simulink model "V10MODE_TEST"  (R2020b)
settings: Solver=VariableStepAuto  StartTime=0.0  StopTime=10.0  RelTol=1e-3
values from neighbouring files (symbols this model uses):
  HD = 180/pi    (= 57.2957795131)    [mode_data.m]
undefined symbols (not defined in the file or in its folder): Vehicle
libraries: sharedutil x2
settings Model: Creator=a4327481  LastModifiedBy=a4327481

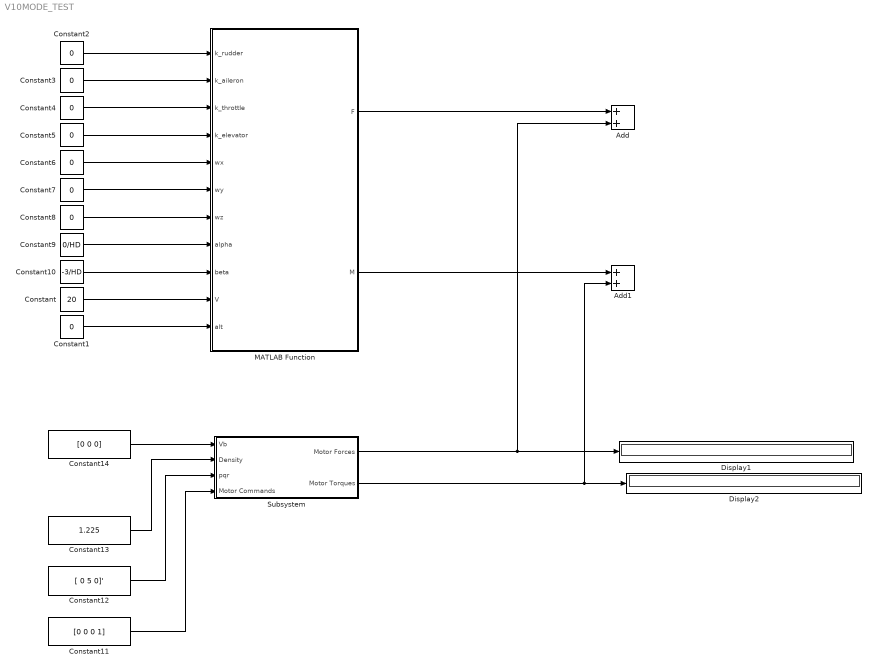
== system V10MODE_TEST ==
  Add : Sum
  Add1 : Sum
  Constant : Constant  Value=20
  Constant{1..8} (8 alike) : Constant  Value=0
  Constant10 : Constant  Value=-3/HD
  Constant11 : Constant  Value=[0 0 0 1]  VectorParams1D=off
  Constant12 : Constant  Value=[ 0 5 0]'
  Constant13 : Constant  Value=1.225
  Constant14 : Constant  Value=[0 0 0]
  Constant9 : Constant  Value=0/HD
  Display1 : Display
  Display2 : Display
  MATLAB Function : MATLAB Function  TreatAsAtomicUnit=on
  Subsystem : Subsystem
  wires:
  Constant/1 -> MATLAB Function/10(V)
  Constant1/1 -> MATLAB Function/11(alt)
  Constant2/1 -> MATLAB Function/1(k_rudder)
  Constant3/1 -> MATLAB Function/2(k_aileron)
  Constant4/1 -> MATLAB Function/3(k_throttle)
  Constant5/1 -> MATLAB Function/4(k_elevator)
  Constant6/1 -> MATLAB Function/5(wx)
  Constant7/1 -> MATLAB Function/6(wy)
  Constant8/1 -> MATLAB Function/7(wz)
  Constant10/1 -> MATLAB Function/9(beta)
  Constant9/1 -> MATLAB Function/8(alpha)
  Constant11/1 -> Subsystem/4(Motor Commands)
  Constant12/1 -> Subsystem/3(pqr)
  Constant13/1 -> Subsystem/2(Density)
  Constant14/1 -> Subsystem/1(Vb)
  MATLAB Function/1(F) -> Add/1
  MATLAB Function/2(M) -> Add1/1
  Subsystem/2(Motor Torques) -> Display2/1, Add1/2
  Subsystem/1(Motor Forces) -> Add/2, Display1/1

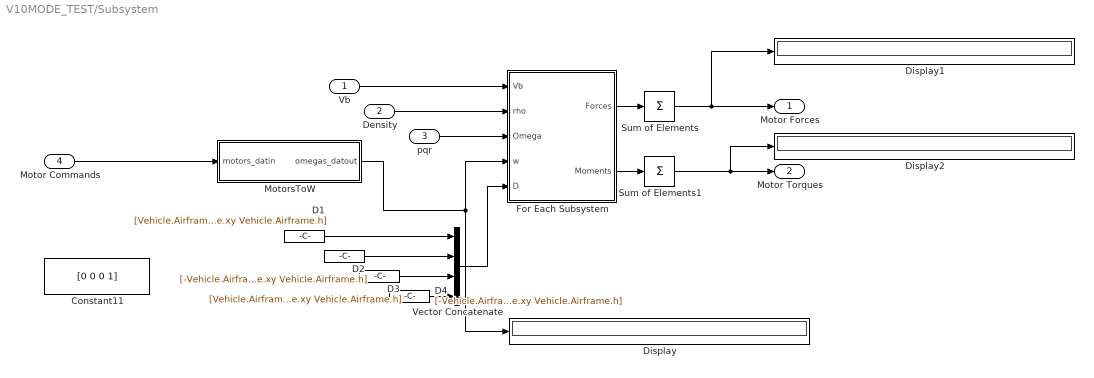
== system V10MODE_TEST/Subsystem ==
  Vb : Inport
  Density : Inport  Port=2
  pqr : Inport  Port=3
  Motor Commands : Inport  Port=4
  Constant11 : Constant  Value=[0 0 0 1]  VectorParams1D=off
  D1 : Constant  Value=[Vehicle.Airframe.xy +Vehicle.Airframe.xy Vehicle.Airframe.h]
  D2 : Constant  Value=[-Vehicle.Airframe.xy -Vehicle.Airframe.xy Vehicle.Airframe.h]
  D3 : Constant  Value=[Vehicle.Airframe.xy -Vehicle.Airframe.xy Vehicle.Airframe.h]
  D4 : Constant  Value=[-Vehicle.Airframe.xy Vehicle.Airframe.xy Vehicle.Airframe.h]
  Display : Display
  Display1 : Display
  Display2 : Display
  For Each Subsystem : Subsystem  TreatAsAtomicUnit=on
  MotorsToW : Subsystem
  Sum of Elements : Sum  Inputs=+  CollapseMode=Specified dimension  CollapseDim=2
  Sum of Elements1 : Sum  Inputs=+  CollapseMode=Specified dimension  CollapseDim=2
  Vector Concatenate : Concatenate  NumInputs=4  Mode=Multidimensional array  ConcatenateDimension=2
  Motor Forces : Outport  Unit=N  VectorParamsAs1DForOutWhenUnconnected=off
  Motor Torques : Outport  Port=2  Unit=N*m  VectorParamsAs1DForOutWhenUnconnected=off
  wires:
  Vector Concatenate/1 -> For Each Subsystem/5(D)
  Density/1 -> For Each Subsystem/2(rho)
  D4/1 -> Vector Concatenate/4
  Vb/1 -> For Each Subsystem/1(Vb)
  Sum of Elements1/1 -> Motor Torques/1, Display2/1
  D3/1 -> Vector Concatenate/3
  Sum of Elements/1 -> Motor Forces/1, Display1/1
  pqr/1 -> For Each Subsystem/3(Omega)
  D1/1 -> Vector Concatenate/1
  For Each Subsystem/2(Moments) -> Sum of Elements1/1
  For Each Subsystem/1(Forces) -> Sum of Elements/1
  D2/1 -> Vector Concatenate/2
  MotorsToW/1(omegas_datout) -> For Each Subsystem/4(w), Display/1
  Motor Commands/1 -> MotorsToW/1(motors_datin)

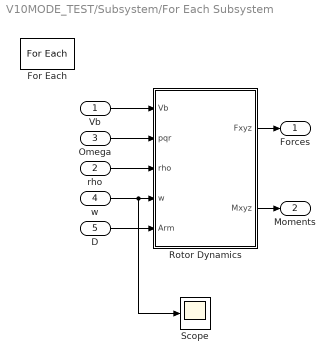
== system V10MODE_TEST/Subsystem/For Each Subsystem ==
  Vb : Inport  PortDimensions=3
  rho : Inport  Port=2  PortDimensions=1
  Omega : Inport  Port=3
  w : Inport  Port=4  Partition=on  PartitionDimension=2  PartitionWidth=1  PartitionOffset=0
  D : Inport  Port=5  Partition=on  PartitionDimension=2  PartitionWidth=1  PartitionOffset=0
  For Each : ForEach  DisableCoverage=on
  Rotor Dynamics : Subsystem  AncestorBlock=dynamicsLibrary/Rotor Dynamics  TreatAsAtomicUnit=on
      mask init:
      | aeroicon('aeroblk');
      settings: RTWFcnNameOpts=Use subsystem name  RTWFileNameOpts=Use function name
  Scope : Scope
  Forces : Outport  ConcatenationDimension=2  VectorParamsAs1DForOutWhenUnconnected=off
  Moments : Outport  Port=2  ConcatenationDimension=2  VectorParamsAs1DForOutWhenUnconnected=off
  wires:
  Rotor Dynamics/1(Fxyz) -> Forces/1
  Rotor Dynamics/2(Mxyz) -> Moments/1
  Vb/1 -> Rotor Dynamics/1(Vb)
  Omega/1 -> Rotor Dynamics/2(pqr)
  rho/1 -> Rotor Dynamics/3(rho)
  D/1 -> Rotor Dynamics/5(Arm)
  w/1 -> Scope/1, Rotor Dynamics/4(w)

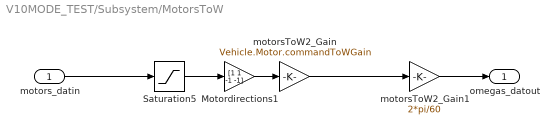
== system V10MODE_TEST/Subsystem/MotorsToW ==
  motors_datin : Inport
  Motordirections1 : Gain  Gain=[1 1 -1 -1]  ParamDataTypeStr=single  OutDataTypeStr=Inherit: Inherit via back propagation  SaturateOnIntegerOverflow=on
  Saturation5 : Saturate  UpperLimit=1  LowerLimit=realmin  OutDataTypeStr=Inherit: Inherit via back propagation
  motorsToW2_Gain : Gain  Gain=Vehicle.Motor.commandToWGain  ParamDataTypeStr=single  OutDataTypeStr=Inherit: Inherit via back propagation  SaturateOnIntegerOverflow=on
  motorsToW2_Gain1 : Gain  Gain=2*pi/60  ParamDataTypeStr=single  OutDataTypeStr=Inherit: Inherit via back propagation  SaturateOnIntegerOverflow=on
  omegas_datout : Outport  VectorParamsAs1DForOutWhenUnconnected=off
  wires:
  Saturation5/1 -> Motordirections1/1
  Motordirections1/1 -> motorsToW2_Gain/1
  motors_datin/1 -> Saturation5/1
  motorsToW2_Gain/1 -> motorsToW2_Gain1/1
  motorsToW2_Gain1/1 -> omegas_datout/1

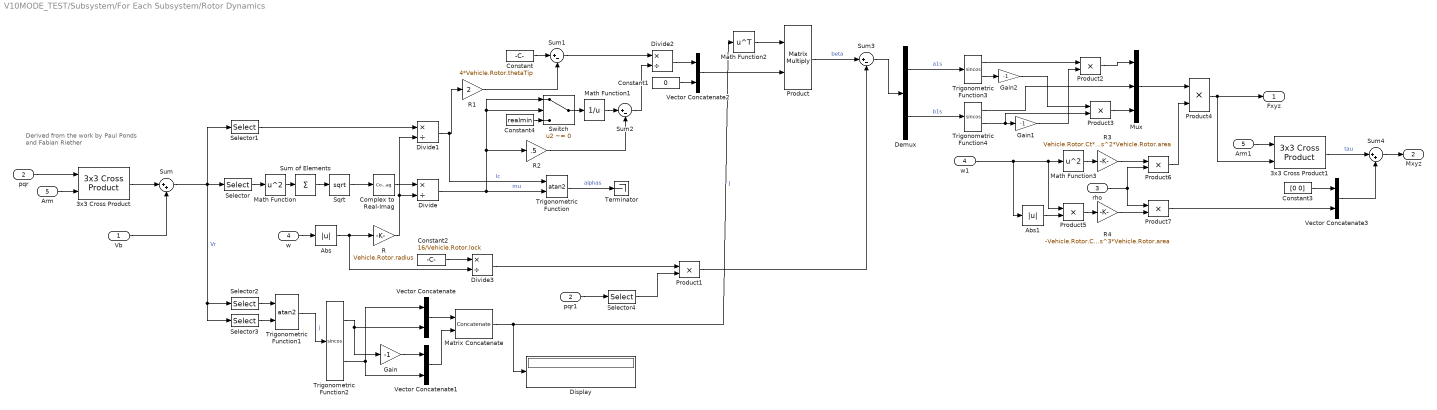
== system V10MODE_TEST/Subsystem/For Each Subsystem/Rotor Dynamics ==
  note: Derived from the work by Paul Ponds
      | and Fabian Riether
  Vb : Inport  PortDimensions=3
  pqr : Inport  Port=2  PortDimensions=3
  rho : Inport  Port=3  PortDimensions=1
  w : Inport  Port=4  PortDimensions=[1 1]
  Arm : Inport  Port=5  PortDimensions=[3 1]
  3x3 Cross Product : sharedutil/3x3 Cross Product  aMode=aMode
      settings: SourceProductBaseCode=AE,PW,MT,UV,VE,VP
  3x3 Cross Product1 : sharedutil/3x3 Cross Product  aMode=aMode
      settings: SourceProductBaseCode=AE,PW,MT,UV,VE,VP
  Abs : Abs
  Abs1 : Abs
  Arm1 : InportShadow  Port=5  PortDimensions=[3 1]
  Complex to Real-Imag : ComplexToRealImag  Output=Real
  Constant : Constant  Value=4*Vehicle.Rotor.thetaTip
  Constant1 : Constant  Value=0
  Constant2 : Constant  Value=16/Vehicle.Rotor.lock
  Constant3 : Constant  Value=[0 0]
  Constant4 : Constant  Value=realmin
  Demux : Demux  Outputs=2
  Display : Display
  Divide{,1..3} (4 alike) : Product  Inputs=*/
  Gain : Gain  Gain=-1
  Gain1 : Gain  Gain=-1
  Gain2 : Gain  Gain=-1
  Math Function : Math  Operator=square  SignedPower=on  SaturateOnIntegerOverflow=on
  Math Function1 : Math  Operator=reciprocal  SignedPower=on  SaturateOnIntegerOverflow=on
  Math Function2 : Math  Operator=transpose  SignedPower=on  SaturateOnIntegerOverflow=on
  Math Function3 : Math  Operator=square  SignedPower=on  SaturateOnIntegerOverflow=on
  Matrix Concatenate : Concatenate  Mode=Multidimensional array  ConcatenateDimension=2
  Mux : Mux  Inputs=3
  Product : Product  Multiplication=Matrix(*)
  Product{1..7} (7 alike) : Product
  R : Gain  Gain=Vehicle.Rotor.radius
  R1 : Gain  Gain=2
  R2 : Gain  Gain=.5
  R3 : Gain  Gain=Vehicle.Rotor.Ct*Vehicle.Rotor.radius^2*Vehicle.Rotor.area
  R4 : Gain  Gain=-Vehicle.Rotor.Cq*Vehicle.Rotor.radius^3*Vehicle.Rotor.area
  Selector : Selector  InputPortWidth=3  IndexOptions=Index vector (dialog)  Indices=[1 2]  OutputSizes=1
  Selector1 : Selector  InputPortWidth=3  IndexOptions=Index vector (dialog)  Indices=[3]  OutputSizes=1
  Selector2 : Selector  InputPortWidth=3  IndexOptions=Index vector (dialog)  Indices=[2]  OutputSizes=1
  Selector3 : Selector  InputPortWidth=3  IndexOptions=Index vector (dialog)  Indices=[1]  OutputSizes=1
  Selector4 : Selector  InputPortWidth=3  IndexOptions=Index vector (dialog)  Indices=[2 1]  OutputSizes=1
  Sqrt : Sqrt  OutputSignalType=complex  SaturateOnIntegerOverflow=on
  Sum : Sum  Inputs=|++
  Sum of Elements : Sum  Inputs=+
  Sum1 : Sum  Inputs=|+-
  Sum2 : Sum  Inputs=|+-
  Sum3 : Sum  Inputs=|+-
  Sum4 : Sum  Inputs=|++
  Switch : Switch  Criteria=u2 ~= 0
  Terminator : Terminator
  Trigonometric Function : Trigonometry  Operator=atan2
  Trigonometric Function1 : Trigonometry  Operator=atan2
  Trigonometric Function2 : Trigonometry  Operator=sincos
  Trigonometric Function3 : Trigonometry  Operator=sincos
  Trigonometric Function4 : Trigonometry  Operator=sincos
  Vector Concatenate{,1..3} (4 alike) : Concatenate
  pqr1 : InportShadow  Port=2  PortDimensions=3
  w1 : InportShadow  Port=4  PortDimensions=[1 1]
  Fxyz : Outport  PortDimensions=[3 1]  VectorParamsAs1DForOutWhenUnconnected=off
  Mxyz : Outport  Port=2  PortDimensions=[3 1]  VectorParamsAs1DForOutWhenUnconnected=off
  wires:
  Complex to Real-Imag/1 -> Divide/1
  Sqrt/1 -> Complex to Real-Imag/1
  Constant4/1 -> Switch/3
  Switch/1 -> Math Function1/1
  Product1/1 -> Sum3/2
  rho/1 -> Product7/1, Product6/2
  Product7/1 -> Vector Concatenate3/2
  Product6/1 -> Product4/2
  Sum4/1 -> Mxyz/1
  3x3 Cross Product1/1 -> Sum4/1  "tau"
  Product4/1 -> Fxyz/1, 3x3 Cross Product1/2
  Arm1/1 -> 3x3 Cross Product1/1
  Vector Concatenate3/1 -> Sum4/2
  Constant3/1 -> Vector Concatenate3/1
  R4/1 -> Product7/2
  Product5/1 -> R4/1
  Abs1/1 -> Product5/2
  R3/1 -> Product6/1
  Mux/1 -> Product4/1
  Gain2/1 -> Product3/1
  Product3/1 -> Mux/3
  Trigonometric Function3/2 -> Gain2/1
  Trigonometric Function4/1 -> Mux/2
  Product2/1 -> Mux/1
  Trigonometric Function3/1 -> Product2/1
  Gain1/1 -> Product2/2
  Trigonometric Function4/2 -> Gain1/1, Product3/2
  Demux/2 -> Trigonometric Function4/1  "b1s"
  Demux/1 -> Trigonometric Function3/1  "a1s"
  Sum3/1 -> Demux/1
  Math Function3/1 -> R3/1
  w1/1 -> Math Function3/1, Product5/1, Abs1/1
  Divide3/1 -> Product1/1
  Abs/1 -> R/1, Divide3/2
  Selector4/1 -> Product1/2
  pqr1/1 -> Selector4/1
  Constant2/1 -> Divide3/1
  Product/1 -> Sum3/1  "beta"
  Math Function2/1 -> Product/1
  Vector Concatenate2/1 -> Product/2
  Constant1/1 -> Vector Concatenate2/2
  Divide2/1 -> Vector Concatenate2/1
  Sum2/1 -> Divide2/2
  R2/1 -> Sum2/2
  Math Function1/1 -> Sum2/1
  Sum1/1 -> Divide2/1
  R1/1 -> Sum1/2
  Constant/1 -> Sum1/1
  Matrix Concatenate/1 -> Display/1, Math Function2/1  "J"
  Vector Concatenate1/1 -> Matrix Concatenate/2
  Vector Concatenate/1 -> Matrix Concatenate/1
  Trigonometric Function2/1 -> Gain/1, Vector Concatenate/2
  Gain/1 -> Vector Concatenate1/1
  Trigonometric Function2/2 -> Vector Concatenate/1, Vector Concatenate1/2
  Trigonometric Function1/1 -> Trigonometric Function2/1  "j"
  Selector3/1 -> Trigonometric Function1/2
  Selector2/1 -> Trigonometric Function1/1
  Trigonometric Function/1 -> Terminator/1  "alphas"
  Divide1/1 -> Trigonometric Function/1, R1/1  "lc"
  Selector1/1 -> Divide1/1
  Divide/1 -> Trigonometric Function/2, Switch/1, Switch/2, R2/1  "mu"
  R/1 -> Divide/2, Divide1/2
  w/1 -> Abs/1
  Arm/1 -> 3x3 Cross Product/2
  pqr/1 -> 3x3 Cross Product/1
  Sum of Elements/1 -> Sqrt/1
  Math Function/1 -> Sum of Elements/1
  Selector/1 -> Math Function/1
  Sum/1 -> Selector/1, Selector1/1, Selector2/1, Selector3/1  "Vr"
  Vb/1 -> Sum/2
  3x3 Cross Product/1 -> Sum/1

== matlab function V10MODE_TEST/MATLAB Function ==
  data: k_rudder input; k_aileron input; k_throttle input; k_elevator input; wx input; wy input; wz input; alpha input; beta input; V input; alt input; Aero parameter; F output; M output
function [F,M] = fcn(k_rudder,k_aileron,k_throttle,k_elevator,wx,wy,wz,alpha,beta,V,alt, Aero)
% 
HD=180/pi;
[~,~,rho,~] = atom_mode(alt+2000);
rho=1.225;
if(V<=5)
    V=0;
end
q=0.5*rho*V*V;
alpha=constrain_value(alpha,-10/HD,12/HD);
beta=constrain_value(beta,-10/HD,12/HD);
Sbw=[cos(alpha)*cos(beta)   -cos(alpha)*sin(beta)   -sin(alpha)
    sin(beta)               cos(beta)               0
    sin(alpha)*cos(beta)    -sin(alpha)*sin(beta)   cos(alpha)];
alpha=alpha*HD;
beta =beta* HD;
CL=interp1(Aero.CL_alpha,Aero.CL,alpha);
CD=interp1(Aero.CD_alpha,Aero.CD,alpha);
CC_beta=interp1(Aero.CC_beta,Aero.CC,abs(beta))*sign(beta);
CC=CC_beta+Aero.CC_dr*k_rudder;
D=q*Aero.Sref*CD;
C=q*Aero.Sref*CC;
L=q*Aero.Sref*CL;
Fw=[D; C; L];
Fb=Sbw*-Fw;
TF=k_throttle*Aero.Tmax;
F_Plane=Fb+[TF;0;0];
%%%%%%%%%%%%%%%%%%%%%%%%%%%%%%%%%%%%%%%%%%%%%%%%%%%%%%%%
Cm_V=interp1(Aero.Cm_alpha,Aero.Cm_V,alpha);
Cm_H=interp1(Aero.Cm_alpha,Aero.Cm_H,alpha);
Cm_L=interp1(Aero.Cm_alpha,Aero.Cm_L,alpha);
Cm_F=interp1(Aero.Cm_alpha,Aero.Cm_F,alpha);
Cm_H_de=interp1(Aero.Cm_elevator,Aero.Cm_H_de,k_elevator);
Cm=Cm_V+Cm_H+Cm_L+Cm_F+Cm_H_de;

Cl_beta=interp1(Aero.beta,Aero.Cl_beta,abs(beta))*sign(beta);
Cl_da=Aero.Cl_da*k_aileron;
Cl=Cl_beta+Cl_da;

Cn_beta=interp1(Aero.beta,Aero.Cn_beta,abs(beta))*sign(beta);
Cn_dr=Aero.Cn_dr*k_rudder;
Cn=Cn_beta+Cn_dr;

l=q*Aero.Sref*Aero.Lref*Cl-0.1*wx;
m=q*Aero.Sref*Aero.Lref*Cm-0.2*wy;
n=q*Aero.Sref*Aero.Lref*Cn-0.2*wz;
M_Plane=[l ;m ;n];

F=F_Plane;
M=M_Plane;

end
